simulink library "CryoDetLibCMB"  (R2016b)
settings: Solver=VariableStepAuto  StartTime=0.0  StopTime=10.0  RelTol=1e-3
undefined symbols (not defined in the file): A, B, C, D, Fadc, Fclk, PCIN, xlipgetpartsetting
libraries: xbsIndex_r4 x640, CryoDetLibCMB x81, CryoDetLib x2, simulink x1
(part 10 of 12)

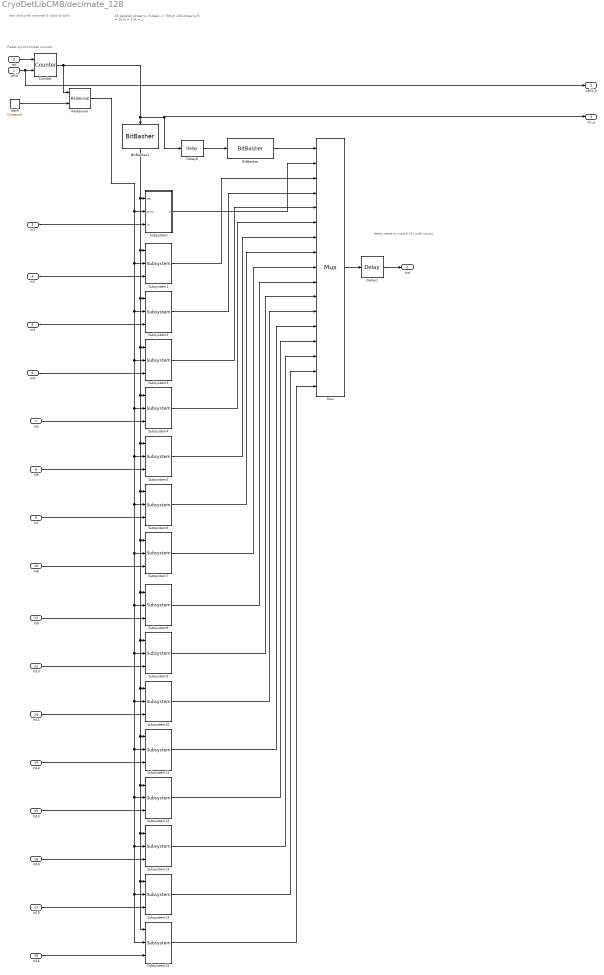
== system CryoDetLibCMB/decimate_128 ==
  note: 16 parallel streams, 8 deep -> TMUX 128 streams
      | R = 16
      | N = 3
      | M = 1
  note: Reset synchronizes counter
  note: set valid with channel 0 valid to sync
  note: delay need to match CH with inputs
  valid : Inport
  rst : Inport  Port=2
  In1 : Inport  Port=3
  In2 : Inport  Port=4
  In3 : Inport  Port=5
  In4 : Inport  Port=6
  In5 : Inport  Port=7
  In6 : Inport  Port=8
  In7 : Inport  Port=9
  In8 : Inport  Port=10
  In9 : Inport  Port=11
  In10 : Inport  Port=12
  In11 : Inport  Port=13
  In12 : Inport  Port=14
  In13 : Inport  Port=15
  In14 : Inport  Port=16
  In15 : Inport  Port=17
  In16 : Inport  Port=18
  BitBasher : xbsIndex_r4/BitBasher  bitexpr=sel = {cnt[3:0]}  display_expr=on  sr_1=sel  arith_type1=Unsigned  bin_pt1=0  sr_2=2  arith_type2=Unsigned  bin_pt2=0  sr_3=3  arith_type3=Unsigned  bin_pt3=0  sr_4=4  arith_type4=Unsigned  bin_pt4=0  dbl_ovrd=off  block_type=bitbasher
  BitBasher1 : xbsIndex_r4/BitBasher  bitexpr=sel = {cnt[6:4]}  display_expr=on  sr_1=sel  arith_type1=Unsigned  bin_pt1=0  sr_2=2  arith_type2=Unsigned  bin_pt2=0  sr_3=3  arith_type3=Unsigned  bin_pt3=0  sr_4=4  arith_type4=Unsigned  bin_pt4=0  dbl_ovrd=off  block_type=bitbasher
  Counter : xbsIndex_r4/Counter  cnt_type=Free Running  cnt_to=Inf  operation=Up  start_count=0  cnt_by_val=1  arith_type=Unsigned  n_bits=7  bin_pt=0  load_pin=off  rst=on  en=on  explicit_period=on  period=2/Fadc  use_behavioral_HDL=off  implementation=Fabric  dbl_ovrd=off  block_type=counter
  Delay1 : xbsIndex_r4/Delay  rst=off  infoeditControl=Selection of Reset will increase slice count due to use of real FFs and instead of SRLs  en=off  latency=14  reg_retiming=on  dbl_ovrd=off  block_type=delay
  Delay6 : xbsIndex_r4/Delay  rst=off  infoeditControl=Selection of Reset will increase slice count due to use of real FFs and instead of SRLs  en=off  latency=1  reg_retiming=on  dbl_ovrd=off  block_type=delay
  Mux : xbsIndex_r4/Mux  inputs=16  en=off  latency=1  precision=Full  arith_type=Unsigned  n_bits=16  bin_pt=14  quantization=Truncate  overflow=Wrap  dbl_ovrd=off  block_type=mux
  Relational : xbsIndex_r4/Relational  mode=a=b  op_type=Bool  en=off  latency=1  dbl_ovrd=off  block_type=relational
  Subsystem : Subsystem
  Subsystem{1..15} (15 alike) : CryoDetLibCMB/decimate_128/Subsystem
  latch : xbsIndex_r4/Constant  const=0  gui_display_data_type=Fixed-point  arith_type=Unsigned  n_bits=7  bin_pt=0  preci_type=Single  exp_width=8  frac_width=24  explicit_period=on  period=2/Fadc  equ=P=C  opselect=C  inp2=PCIN>>17  opr=+  inp1=P  carry=CIN  dbl_ovrd=off  block_type=constant
  valid_o : Outport
  out : Outport  Port=2
  ch_o : Outport  Port=3
  wires:
  rst/1 -> Counter/1
  Delay1/1 -> out/1
  valid/1 -> Counter/2, valid_o/1
  BitBasher1/1 -> Subsystem/1(sel), Subsystem1/1, Subsystem2/1, Subsystem3/1, Subsystem4/1, Subsystem5/1, Subsystem6/1, Subsystem7/1, Subsystem8/1, Subsystem9/1, Subsystem10/1, Subsystem11/1, Subsystem12/1, Subsystem13/1, Subsystem15/1, Subsystem14/1
  Counter/1 -> BitBasher1/1, Delay6/1, ch_o/1, Relational/1
  Subsystem3/1 -> Mux/5
  Mux/1 -> Delay1/1
  In16/1 -> Subsystem15/3
  In15/1 -> Subsystem14/3
  In14/1 -> Subsystem13/3
  In13/1 -> Subsystem12/3
  In12/1 -> Subsystem11/3
  In11/1 -> Subsystem10/3
  In10/1 -> Subsystem9/3
  In9/1 -> Subsystem8/3
  In8/1 -> Subsystem7/3
  In7/1 -> Subsystem6/3
  In6/1 -> Subsystem5/3
  In5/1 -> Subsystem4/3
  In4/1 -> Subsystem3/3
  In3/1 -> Subsystem2/3
  In2/1 -> Subsystem1/3
  In1/1 -> Subsystem/3(in)
  Subsystem15/1 -> Mux/17
  Subsystem14/1 -> Mux/16
  Subsystem13/1 -> Mux/15
  Subsystem12/1 -> Mux/14
  Subsystem11/1 -> Mux/13
  Subsystem10/1 -> Mux/12
  Subsystem9/1 -> Mux/11
  Subsystem8/1 -> Mux/10
  Subsystem7/1 -> Mux/9
  Subsystem6/1 -> Mux/8
  Subsystem5/1 -> Mux/7
  Subsystem4/1 -> Mux/6
  Subsystem2/1 -> Mux/4
  Subsystem1/1 -> Mux/3
  Subsystem/1(o) -> Mux/2
  BitBasher/1 -> Mux/1
  Relational/1 -> Subsystem/2(sync), Subsystem1/2, Subsystem2/2, Subsystem3/2, Subsystem4/2, Subsystem5/2, Subsystem6/2, Subsystem7/2, Subsystem8/2, Subsystem9/2, Subsystem10/2, Subsystem11/2, Subsystem12/2, Subsystem13/2, Subsystem15/2, Subsystem14/2
  latch/1 -> Relational/2
  Delay6/1 -> BitBasher/1

== system CryoDetLibCMB/demod 8Ch ==
  note: Scale by channel amplitude
  note: not tested yet!!!
  note: check scope for tlast errors
  note: Unity gain scaling is 2^-12
      | Here we add factor of 8 gain
      | assuming no single line is grater than -18 dBfs on ADC
  note: Should be 0 if prop delays adjusted properl
  note: compare subBand numbers to test for proper latency
      | diff should be zero otherwise adjust delay of suBand number to DDS block
  note: decimate by 16 3rd order
      | and adjust scaling appropriately
  note: Downconverter
  note: Multiply complex Signal & Reference
      | by complex LO and lowpass filter
      | send complex LO to:
      | 	DAC out
      | 	reference phase
      | ID is which demodulator is this one
  note: break out complex ADC signal
      | multiply by appropriate complex LO
      | then CIC decimate by 16
  note: first data comes out XX ticks after release of reset
  ID : Inport
  freqBus : Inport  Port=2
  In : Inport  Port=3
  amplBus : Inport  Port=4
  AddSub : xbsIndex_r4/AddSub  mode=Subtraction  use_carryin=off  use_carryout=off  en=off  latency=1  precision=User Defined  arith_type="Signed  (2's comp)"  n_bits=3  bin_pt=0  quantization=Truncate  overflow=Wrap  use_behavioral_HDL=off  hw_selection=Fabric  pipelined=off  dbl_ovrd=off  block_type=addsub
  Bus Creator1 : BusCreator  Inputs=4
  Bus Selector1 : BusSelector  OutputSignals=INDX,Q,I
  Bus Selector2 : BusSelector  OutputSignals=INDX,Q,I
  "CIC Compiler 4.0 " : xbsIndex_r4/CIC Compiler 4.0   filter_type=Decimation  number_of_stages=3  differential_delay=1  number_of_channels=8  sample_rate_changes=Fixed  fixed_or_initial_rate=16  minimum_rate=16  maximum_rate=16  ratespecification=Sample_Period  sampleperiod=1  hardwareoversamplingrate=1  quantization=Truncation  output_data_width=20  use_xtreme_dsp_slice=off  use_streaming_interface=on  has_aclken=off  has_aresetn=on  has_dout_tready=off  trim_axipin_name=on  gui_behaviour=Sysgen_GUI  input_data_width=18  ip_name=CIC Compiler  ip_version=4.0  dsptool_ready=true  wrapper_available=true  port_translation_map={ 'aclken' => 'en', 'aresetn' => 'rst' }  ipcore_xco_need_fpga_part=true  ipcore_verbose=false  block_type=cic_compiler_v4_0
  CIC Compiler 4.0 1 : xbsIndex_r4/CIC Compiler 4.0   filter_type=Decimation  number_of_stages=3  differential_delay=1  number_of_channels=8  sample_rate_changes=Fixed  fixed_or_initial_rate=16  minimum_rate=16  maximum_rate=16  ratespecification=Sample_Period  sampleperiod=1  hardwareoversamplingrate=1  quantization=Truncation  output_data_width=20  use_xtreme_dsp_slice=off  use_streaming_interface=on  has_aclken=off  has_aresetn=on  has_dout_tready=off  trim_axipin_name=on  gui_behaviour=Sysgen_GUI  input_data_width=18  ip_name=CIC Compiler  ip_version=4.0  dsptool_ready=true  wrapper_available=true  port_translation_map={ 'aclken' => 'en', 'aresetn' => 'rst' }  ipcore_xco_need_fpga_part=true  ipcore_verbose=false  block_type=cic_compiler_v4_0
  CIC debug scope : Scope  NumInputPorts=3
  CIC reset : Subsystem
  "Complex Multiplier 6.0 " : xbsIndex_r4/Complex Multiplier 6.0   hasatlast=off  hasatuser=on  atuserwidth=3  hasbtlast=off  hasbtuser=off  btuserwidth=1  multtype=Use_Mults  optimizegoal=Resources  flowcontrol=NonBlocking  outputwidth=18  roundmode=Truncate  hasctrltlast=off  hasctrltuser=off  ctrltuserwidth=1  outtlastbehv=Null  latencyconfig=Manual  minimumlatency=6  aclken=off  aresetn=off  trim_axipin_name=on  simulation_type=hybrid_sim  simulation_model=sysgen:cmpy_v6_0  data_path_portlist={ 's_axis_a_tdata_real', 's_axis_a_tdata_imag', 's_axis_b_tdata_real', 's_axis_b_tdata_imag', 's_axis_ctrl_tdata_rounding_bit', 'm_axis_dout_tdata_real', 'm_axis_dout_tdata_imag' }  aportwidth=63  bportwidth=63  ip_name=Complex Multiplier  ip_version=6.0  dsptool_ready=true  ipcore_usecache=true  ipcore_useipmodelcache=true  ipcore_verbose=false  ipcore_latency_parameter='minimumlatency'  wrapper_available=true  port_translation_map={ 'aclken' => 'en', 'aresetn' => 'rst'}  block_type=cmpy_v6_0
  Constant : xbsIndex_r4/Constant  const=1  gui_display_data_type=Boolean  arith_type=Boolean  n_bits=16  bin_pt=14  preci_type=Single  exp_width=8  frac_width=24  explicit_period=off  period=1  equ=P=C  opselect=C  inp2=PCIN>>17  opr=+  inp1=P  carry=CIN  dbl_ovrd=off  block_type=constant
  Constant1 : xbsIndex_r4/Constant  const=1  gui_display_data_type=Boolean  arith_type=Boolean  n_bits=16  bin_pt=14  preci_type=Single  exp_width=8  frac_width=24  explicit_period=off  period=1  equ=P=C  opselect=C  inp2=PCIN>>17  opr=+  inp1=P  carry=CIN  dbl_ovrd=off  block_type=constant
  Constant4 : xbsIndex_r4/Constant  const=14  gui_display_data_type=Fixed-point  arith_type=Unsigned  n_bits=4  bin_pt=0  preci_type=Single  exp_width=8  frac_width=24  explicit_period=off  period=1  equ=P=C  opselect=C  inp2=PCIN>>17  opr=+  inp1=P  carry=CIN  dbl_ovrd=off  block_type=constant
  DDS 8ch : Subsystem
  Delay1 : xbsIndex_r4/Delay  rst=off  infoeditControl=Selection of Reset will increase slice count due to use of real FFs and instead of SRLs  en=off  latency=1  reg_retiming=on  dbl_ovrd=off  block_type=delay
  Delay5 : xbsIndex_r4/Delay  rst=off  infoeditControl=Selection of Reset will increase slice count due to use of real FFs and instead of SRLs  en=off  latency=1  reg_retiming=on  dbl_ovrd=off  block_type=delay
  Delay6 : xbsIndex_r4/Delay  rst=off  infoeditControl=Selection of Reset will increase slice count due to use of real FFs and instead of SRLs  en=off  latency=1  reg_retiming=on  dbl_ovrd=off  block_type=delay
  Display : Display
  Gateway Out{,1..5} (6 alike) : xbsIndex_r4/Gateway Out  inherit_from_input=off  hdl_port=off  rows=1  columns=1  UseAsDAC=off  DACChannel='1'  interface=None  automatic_assignment=on  address_offset=hex2dec('00')  intf_name=''  intf_description=''  timing_constraint=None  locs_specified=off  LOCs={}  io_standard={}  block_type=gatewayout
  Mux : Mux  Inputs=2
  Mux1 : Mux  Inputs=2
  Scale1 : xbsIndex_r4/Scale  scale_factor=-9  dbl_ovrd=off  block_type=scale
  Scale2 : xbsIndex_r4/Scale  scale_factor=-9  dbl_ovrd=off  block_type=scale
  Set Ampls : Subsystem
  Terminator1 : Terminator
  Terminator2 : Terminator
  Terminator3 : Terminator
  phaseRefDownsample : Subsystem
  demod : Outport
  phase ref : Outport  Port=2
  tones out : Outport  Port=3
  wires:
  In/1 -> Bus Selector2/1
  Bus Selector1/2 -> "Complex Multiplier 6.0 "/2  "<Q>"
  Bus Selector1/3 -> "Complex Multiplier 6.0 "/3  "<I>"
  "Complex Multiplier 6.0 "/2 -> "CIC Compiler 4.0 "/2
  "CIC Compiler 4.0 "/3 -> Scale1/1
  CIC Compiler 4.0 1/3 -> Scale2/1
  "CIC Compiler 4.0 "/1 -> Terminator1/1
  CIC Compiler 4.0 1/1 -> Terminator2/1
  CIC Compiler 4.0 1/2 -> Terminator3/1
  "Complex Multiplier 6.0 "/3 -> CIC Compiler 4.0 1/2
  Constant/1 -> "Complex Multiplier 6.0 "/5, "Complex Multiplier 6.0 "/1
  ID/1 -> DDS 8ch/1(ID), [ID]
  freqBus/1 -> DDS 8ch/2(freqBus)
  Bus Selector2/1 -> Delay1/1, DDS 8ch/3(band)  "<INDX>"
  Bus Selector2/2 -> Delay5/1  "<Q>"
  Bus Selector2/3 -> Delay6/1  "<I>"
  DDS 8ch/1(IQ out) -> tones out/1, Bus Selector1/1
  Delay1/1 -> AddSub/2, "Complex Multiplier 6.0 "/4
  Delay5/1 -> "Complex Multiplier 6.0 "/6
  Delay6/1 -> "Complex Multiplier 6.0 "/7
  Bus Selector1/1 -> AddSub/1  "<INDX>"
  AddSub/1 -> Gateway Out/1
  Gateway Out/1 -> Display/1
  Constant1/1 -> CIC Compiler 4.0 1/1, "CIC Compiler 4.0 "/1
  Constant4/1 -> CIC reset/3(N-2)
  [fpgaReset] -> CIC reset/1(resetIn)
  CIC reset/1(notResetOut) -> "CIC Compiler 4.0 "/4, CIC Compiler 4.0 1/4
  "Complex Multiplier 6.0 "/4 -> CIC reset/2(Channel)
  CIC reset/2(tlast) -> CIC Compiler 4.0 1/3, "CIC Compiler 4.0 "/3
  "CIC Compiler 4.0 "/6 -> Bus Creator1/2  "band"
  Scale1/1 -> Bus Creator1/3  "Q"
  Scale2/1 -> Bus Creator1/4  "I"
  CIC Compiler 4.0 1/4 -> Gateway Out1/1
  CIC Compiler 4.0 1/5 -> phaseRefDownsample/2(chanSynch), Gateway Out2/1
  CIC Compiler 4.0 1/6 -> Gateway Out3/1
  CIC Compiler 4.0 1/7 -> Gateway Out4/1
  CIC Compiler 4.0 1/8 -> Gateway Out5/1
  Gateway Out2/1 -> Mux/2
  Gateway Out1/1 -> Mux/1
  Gateway Out5/1 -> Mux1/2
  Gateway Out4/1 -> Mux1/1
  Mux/1 -> CIC debug scope/1
  Gateway Out3/1 -> CIC debug scope/2
  Mux1/1 -> CIC debug scope/3
  "CIC Compiler 4.0 "/2 -> Bus Creator1/1  "tvalid"
  DDS 8ch/2(phaseRef out) -> phaseRefDownsample/1(In1)
  phaseRefDownsample/1(Out1) -> phase ref/1
  Bus Creator1/1 -> Set Ampls/3(DDS IQ)
  Set Ampls/1(IQ out) -> demod/1
  [ID] -> Set Ampls/1(ID)
  amplBus/1 -> Set Ampls/2(amplBus)

== system CryoDetLibCMB/demod setup stuff ==
  Bus Creator : BusCreator  Inputs=3
  Bus Creator1 : BusCreator  Inputs=3
  Counter Free-Running1 : simulink/Sources/Counter Free-Running  NumBits=3  tsamp=Tclk
  I : xbsIndex_r4/Constant  const=1  gui_display_data_type=Fixed-point  arith_type=Signed (2's comp)  n_bits=25  bin_pt=24  preci_type=Single  exp_width=8  frac_width=24  explicit_period=on  period=Tclk  equ=P=C  opselect=C  inp2=PCIN>>17  opr=+  inp1=P  carry=CIN  dbl_ovrd=off  block_type=constant
  Ndemod : xbsIndex_r4/Constant  const=15  gui_display_data_type=Fixed-point  arith_type=Unsigned  n_bits=4  bin_pt=0  preci_type=Single  exp_width=8  frac_width=24  explicit_period=off  period=1  equ=P=C  opselect=C  inp2=PCIN>>17  opr=+  inp1=P  carry=CIN  dbl_ovrd=off  block_type=constant
  Q : xbsIndex_r4/Constant  const=0  gui_display_data_type=Fixed-point  arith_type=Signed (2's comp)  n_bits=25  bin_pt=24  preci_type=Single  exp_width=8  frac_width=24  explicit_period=on  period=Tclk  equ=P=C  opselect=C  inp2=PCIN>>17  opr=+  inp1=P  carry=CIN  dbl_ovrd=off  block_type=constant
  demod # : xbsIndex_r4/Constant  const=15  gui_display_data_type=Fixed-point  arith_type=Unsigned  n_bits=4  bin_pt=0  preci_type=Single  exp_width=8  frac_width=24  explicit_period=off  period=1  equ=P=C  opselect=C  inp2=PCIN>>17  opr=+  inp1=P  carry=CIN  dbl_ovrd=off  block_type=constant
  freq2 : xbsIndex_r4/Constant  const=0.12345 * 2^24  gui_display_data_type=Fixed-point  arith_type=Unsigned  n_bits=24  bin_pt=0  preci_type=Single  exp_width=8  frac_width=24  explicit_period=on  period=Tclk  equ=P=C  opselect=C  inp2=PCIN>>17  opr=+  inp1=P  carry=CIN  dbl_ovrd=off  block_type=constant
  subCh : xbsIndex_r4/Constant  const=7  gui_display_data_type=Fixed-point  arith_type=Unsigned  n_bits=3  bin_pt=0  preci_type=Single  exp_width=8  frac_width=24  explicit_period=off  period=1  equ=P=C  opselect=C  inp2=PCIN>>17  opr=+  inp1=P  carry=CIN  dbl_ovrd=off  block_type=constant
  demod numberl : Outport
  freqBus : Outport  Port=2
  subBandIQ : Outport  Port=3
  wires:
  Bus Creator/1 -> freqBus/1
  demod #/1 -> demod numberl/1
  freq2/1 -> Bus Creator/3  "freq"
  subCh/1 -> Bus Creator/1  "band"
  Ndemod/1 -> Bus Creator/2  "chan"
  Bus Creator1/1 -> subBandIQ/1
  Counter Free-Running1/1 -> Bus Creator1/1  "INDX"
  Q/1 -> Bus Creator1/2  "Q"
  I/1 -> Bus Creator1/3  "I"

== system CryoDetLibCMB/freqWordDecoder ==
  Fi : Inport
  BitBasher : xbsIndex_r4/BitBasher  bitexpr=|  display_expr=on  sr_1=FBen  arith_type1=Unsigned  bin_pt1=0  sr_2=ampl  arith_type2=Unsigned  bin_pt2=0  sr_3=Finit  arith_type3=Unsigned  bin_pt3=24  sr_4=4  arith_type4=Unsigned  bin_pt4=0  dbl_ovrd=off  block_type=bitbasher
      | FBen = {freqWord[31:31]}
      | ampl = {freqWord[27:24]}
      | Finit = {freqWord[23:0]}
  FBen : Outport
  ampl : Outport  Port=2
  Fc : Outport  Port=3
  wires:
  BitBasher/2 -> ampl/1
  BitBasher/3 -> Fc/1
  BitBasher/1 -> FBen/1
  Fi/1 -> BitBasher/1

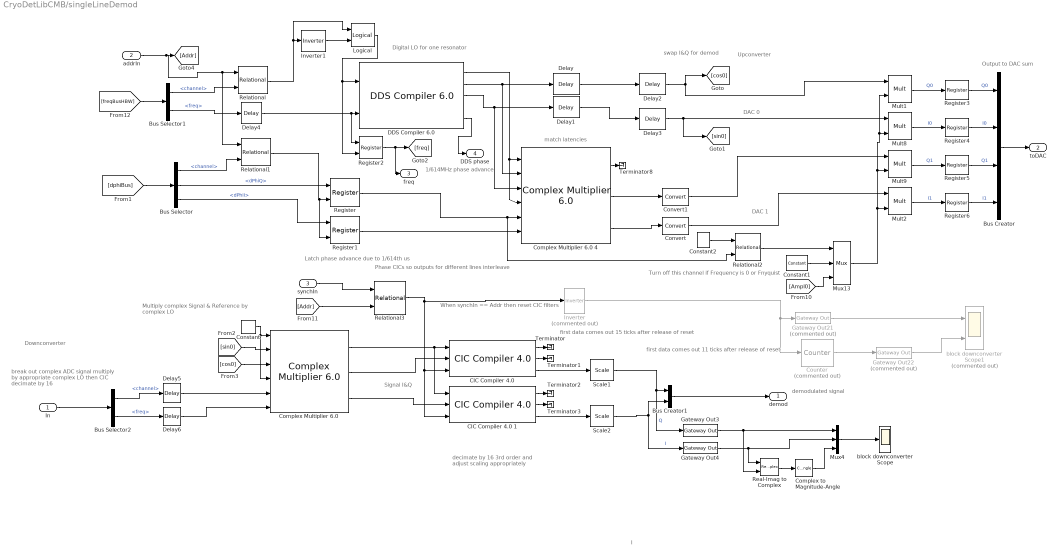
== system CryoDetLibCMB/singleLineDemod ==
  note: swap I&Q for demod
  note: Output to DAC sum
  note: decimate by 16 3rd order
      | and adjust scaling appropriately
  note: When synchIn == Addr then reset CIC filters
  note: Turn off this channel if Frequency is 0 or Fnyquist
  note: first data comes out 15 ticks after release of reset
  note: Latch phase advance due to 1/614th us
  note: I
  note: DAC 1
  note: DAC 0
  note: Downconverter
  note: demodulated signal
  note: Phase CICs so outputs for different lines interleave
  note: Signal I&Q
  note: Multiply complex Signal & Reference
      | by complex LO
  note: match latencies
  note: 1/614MHz
      | phase advance
  note: break out complex ADC signal
      | multiply by appropriate complex LO
      | then CIC decimate by 16
  note: Digital LO for one resonator
  note: Upconverter
  note: first data comes out 11 ticks after release of reset
  In : Inport
  addrIn : Inport  Port=2
  synchIn : Inport  Port=3
  Bus Creator : BusCreator  Inputs=4
  Bus Creator1 : BusCreator  Inputs=2
  Bus Selector : BusSelector  OutputSignals=channel,dPhiQ,dPhiI
  Bus Selector1 : BusSelector  OutputSignals=channel,freq
  Bus Selector2 : BusSelector  OutputSignals=channel,freq
  "CIC Compiler 4.0 " : xbsIndex_r4/CIC Compiler 4.0   filter_type=Decimation  number_of_stages=3  differential_delay=1  number_of_channels=1  sample_rate_changes=Fixed  fixed_or_initial_rate=16  minimum_rate=16  maximum_rate=16  ratespecification=Sample_Period  sampleperiod=1  hardwareoversamplingrate=1  quantization=Truncation  output_data_width=20  use_xtreme_dsp_slice=off  use_streaming_interface=on  has_aclken=off  has_aresetn=on  has_dout_tready=off  trim_axipin_name=on  gui_behaviour=Sysgen_GUI  input_data_width=18  ip_name=CIC Compiler  ip_version=4.0  dsptool_ready=true  wrapper_available=true  port_translation_map={ 'aclken' => 'en', 'aresetn' => 'rst' }  ipcore_xco_need_fpga_part=true  ipcore_verbose=false  block_type=cic_compiler_v4_0
  CIC Compiler 4.0 1 : xbsIndex_r4/CIC Compiler 4.0   filter_type=Decimation  number_of_stages=3  differential_delay=1  number_of_channels=1  sample_rate_changes=Fixed  fixed_or_initial_rate=16  minimum_rate=16  maximum_rate=16  ratespecification=Sample_Period  sampleperiod=1  hardwareoversamplingrate=1  quantization=Truncation  output_data_width=20  use_xtreme_dsp_slice=off  use_streaming_interface=on  has_aclken=off  has_aresetn=on  has_dout_tready=off  trim_axipin_name=on  gui_behaviour=Sysgen_GUI  input_data_width=18  ip_name=CIC Compiler  ip_version=4.0  dsptool_ready=true  wrapper_available=true  port_translation_map={ 'aclken' => 'en', 'aresetn' => 'rst' }  ipcore_xco_need_fpga_part=true  ipcore_verbose=false  block_type=cic_compiler_v4_0
  "Complex Multiplier 6.0 " : xbsIndex_r4/Complex Multiplier 6.0   hasatlast=off  hasatuser=off  atuserwidth=1  hasbtlast=off  hasbtuser=off  btuserwidth=1  multtype=Use_Mults  optimizegoal=Resources  flowcontrol=NonBlocking  outputwidth=18  roundmode=Truncate  hasctrltlast=off  hasctrltuser=off  ctrltuserwidth=1  outtlastbehv=Null  latencyconfig=Automatic  minimumlatency=37  aclken=off  aresetn=off  trim_axipin_name=on  simulation_type=hybrid_sim  simulation_model=sysgen:cmpy_v6_0  data_path_portlist={ 's_axis_a_tdata_real', 's_axis_a_tdata_imag', 's_axis_b_tdata_real', 's_axis_b_tdata_imag', 's_axis_ctrl_tdata_rounding_bit', 'm_axis_dout_tdata_real', 'm_axis_dout_tdata_imag' }  aportwidth=63  bportwidth=63  ip_name=Complex Multiplier  ip_version=6.0  dsptool_ready=true  ipcore_usecache=true  ipcore_useipmodelcache=true  ipcore_verbose=false  ipcore_latency_parameter='minimumlatency'  wrapper_available=true  port_translation_map={ 'aclken' => 'en', 'aresetn' => 'rst'}  block_type=cmpy_v6_0
  Complex Multiplier 6.0 4 : xbsIndex_r4/Complex Multiplier 6.0   hasatlast=off  hasatuser=off  atuserwidth=1  hasbtlast=off  hasbtuser=off  btuserwidth=1  multtype=Use_Mults  optimizegoal=Resources  flowcontrol=NonBlocking  outputwidth=19  roundmode=Truncate  hasctrltlast=off  hasctrltuser=off  ctrltuserwidth=1  outtlastbehv=Null  latencyconfig=Manual  minimumlatency=6  aclken=off  aresetn=off  trim_axipin_name=on  simulation_type=hybrid_sim  simulation_model=sysgen:cmpy_v6_0  data_path_portlist={ 's_axis_a_tdata_real', 's_axis_a_tdata_imag', 's_axis_b_tdata_real', 's_axis_b_tdata_imag', 's_axis_ctrl_tdata_rounding_bit', 'm_axis_dout_tdata_real', 'm_axis_dout_tdata_imag' }  aportwidth=63  bportwidth=63  ip_name=Complex Multiplier  ip_version=6.0  dsptool_ready=true  ipcore_usecache=true  ipcore_useipmodelcache=true  ipcore_verbose=false  ipcore_latency_parameter='minimumlatency'  wrapper_available=true  port_translation_map={ 'aclken' => 'en', 'aresetn' => 'rst'}  block_type=cmpy_v6_0
  Complex to Magnitude-Angle : ComplexToMagnitudeAngle  Output=Magnitude
  Constant : xbsIndex_r4/Constant  const=1  gui_display_data_type=Boolean  arith_type=Boolean  n_bits=16  bin_pt=14  preci_type=Single  exp_width=8  frac_width=24  explicit_period=off  period=1  equ=P=C  opselect=C  inp2=PCIN>>17  opr=+  inp1=P  carry=CIN  dbl_ovrd=off  block_type=constant
  Constant1 : xbsIndex_r4/Constant  const=0  gui_display_data_type=Fixed-point  arith_type=Unsigned  n_bits=16  bin_pt=16  preci_type=Single  exp_width=8  frac_width=24  explicit_period=off  period=1  equ=P=C  opselect=C  inp2=PCIN>>17  opr=+  inp1=P  carry=CIN  dbl_ovrd=off  block_type=constant
  Constant2 : xbsIndex_r4/Constant  const=0  gui_display_data_type=Fixed-point  arith_type=Unsigned  n_bits=16  bin_pt=16  preci_type=Single  exp_width=8  frac_width=24  explicit_period=off  period=1  equ=P=C  opselect=C  inp2=PCIN>>17  opr=+  inp1=P  carry=CIN  dbl_ovrd=off  block_type=constant
  Convert : xbsIndex_r4/Convert  gui_display_data_type=Fixed-point  arith_type="Signed  (2's comp)"  n_bits=16  bin_pt=14  float_type=Single  exp_bits=8  fraction_bits=24  quantization=Truncate  overflow=Saturate  en=off  latency=1  pipeline=off  dbl_ovrd=off  block_type=convert
  Convert1 : xbsIndex_r4/Convert  gui_display_data_type=Fixed-point  arith_type="Signed  (2's comp)"  n_bits=16  bin_pt=14  float_type=Single  exp_bits=8  fraction_bits=24  quantization=Truncate  overflow=Saturate  en=off  latency=1  pipeline=off  dbl_ovrd=off  block_type=convert
  Counter : xbsIndex_r4/Counter  Commented=on  cnt_type=Free Running  cnt_to=Inf  operation=Up  start_count=0  cnt_by_val=2^-8  arith_type=Unsigned  n_bits=8  bin_pt=8  load_pin=off  rst=on  en=off  explicit_period=off  period=1  use_behavioral_HDL=off  implementation=Fabric  dbl_ovrd=off  block_type=counter
  "DDS Compiler 6.0 " : xbsIndex_r4/DDS Compiler 6.0   partspresent=Phase_Generator_and_SIN_COS_LUT  dds_clock_rate=Fclk/1e6  channels=1  mode_of_operation=Standard  modulus=9  parameter_entry=Hardware_Parameters  spurious_free_dynamic_range=45  frequency_resolution=0.4  noise_shaping=None  phase_width=freqBits  output_width=IQbits  output_selection=Sine_and_Cosine  negative_sine=off  negative_cosine=off  amplitude_mode=Unit_Circle  memory_type=Auto  optimization_goal=Speed  dsp48_use=Maximal  resync=off  latency_configuration=Configurable  latency=15  has_phase_out=on  has_aclken=off  has_aresetn=off  explicit_period=on  period=Tclk  data_has_tlast=Not_Required  has_tready=off  s_phase_has_tuser=Not_Required  m_data_has_tuser=Not_Required  m_phase_has_tuser=Not_Required  s_phase_tuser_width=1  output_form=Twos_Complement  s_config_sync_mode=On_Vector  phase_increment=Programmable  output_frequency1=0  output_frequency2=0  output_frequency3=0  output_frequency4=0  output_frequency5=0  output_frequency6=0  output_frequency7=0  output_frequency8=0  output_frequency9=0  output_frequency10=0  output_frequency11=0  output_frequency12=0  output_frequency13=0  output_frequency14=0  output_frequency15=0  output_frequency16=0  pinc1='0'  pinc2='0'  pinc3='0'  pinc4='0'  pinc5='0'  pinc6='0'  pinc7='0'  pinc8='0'  pinc9='0'  pinc10='0'  pinc11='0'  pinc12='0'  pinc13='0'  pinc14='0'  pinc15='0'  pinc16='0'  phase_offset=None  phase_offset_angles1=0  phase_offset_angles2=0  phase_offset_angles3=0  phase_offset_angles4=0  phase_offset_angles5=0  phase_offset_angles6=0  phase_offset_angles7=0  phase_offset_angles8=0  phase_offset_angles9=0  phase_offset_angles10=0  phase_offset_angles11=0  phase_offset_angles12=0  phase_offset_angles13=0  phase_offset_angles14=0  phase_offset_angles15=0  phase_offset_angles16=0  poff1='0'  poff2='0'  poff3='0'  poff4='0'  poff5='0'  poff6='0'  poff7='0'  poff8='0'  poff9='0'  poff10='0'  poff11='0'  poff12='0'  poff13='0'  poff14='0'  poff15='0'  poff16='0'  trim_axipin_name=on  simulation_type=hybrid_sim  simulation_model=sysgen:xddsv6_0_cmodel  data_path_portlist={ 's_axis_config_tdata_poff', 's_axis_config_tdata_chan0_poff', 's_axis_config_tdata_pinc', 's_axis_config_tdata_chan0_pinc', 's_axis_phase_tdata_resync', 's_axis_phase_tdata_chan0_resync', 's_axis_phase_tdata_poff', 's_axis_phase_tdata_chan0_poff', 's_axis_phase_tdata_pinc', 's_axis_phase_tdata_chan0_pinc', 's_axis_phase_tdata_phase_in', 'm_axis_data_tdata_sine', 'm_axis_data_tdata_chan0_sine', 'm_axis_data_tdata_cosine', 'm_axis_data_tdata_chan0_cosine', 'm_axis_phase_tdata_phase_out', 'm_axis_phase_tdata_chan0_phase_out'}  por_mode=false  gui_behaviour=Sysgen  ip_name=DDS Compiler  ip_version=6.0  dsptool_ready=true  wrapper_available=true  port_translation_map={ 'aclken' => 'en', 'aresetn' => 'rst' }  ipcore_usecache=true  ipcore_useipmodelcache=true  ipcore_xco_need_fpga_part=true  ipcore_fpga_part=xlipgetpartsetting(gcb, {'kintex7', 'xc7k325t', '-3', 'fbg676'})  ipcore_verbose=false  block_type=dds_compiler_v6_0
  Delay : xbsIndex_r4/Delay  rst=off  infoeditControl=Selection of Reset will increase slice count due to use of real FFs and instead of SRLs  en=off  latency=6  reg_retiming=off  dbl_ovrd=off  block_type=delay
  Delay1 : xbsIndex_r4/Delay  rst=off  infoeditControl=Selection of Reset will increase slice count due to use of real FFs and instead of SRLs  en=off  latency=6  reg_retiming=off  dbl_ovrd=off  block_type=delay
  Delay2 : xbsIndex_r4/Delay  rst=off  infoeditControl=Selection of Reset will increase slice count due to use of real FFs and instead of SRLs  en=off  latency=1  reg_retiming=off  dbl_ovrd=off  block_type=delay
  Delay3 : xbsIndex_r4/Delay  rst=off  infoeditControl=Selection of Reset will increase slice count due to use of real FFs and instead of SRLs  en=off  latency=1  reg_retiming=off  dbl_ovrd=off  block_type=delay
  Delay4 : xbsIndex_r4/Delay  rst=off  infoeditControl=Selection of Reset will increase slice count due to use of real FFs and instead of SRLs  en=off  latency=2  reg_retiming=on  dbl_ovrd=off  block_type=delay
  Delay5 : xbsIndex_r4/Delay  rst=off  infoeditControl=Selection of Reset will increase slice count due to use of real FFs and instead of SRLs  en=off  latency=2  reg_retiming=on  dbl_ovrd=off  block_type=delay
  Delay6 : xbsIndex_r4/Delay  rst=off  infoeditControl=Selection of Reset will increase slice count due to use of real FFs and instead of SRLs  en=off  latency=2  reg_retiming=on  dbl_ovrd=off  block_type=delay
  Gateway Out21 : xbsIndex_r4/Gateway Out  Commented=on  inherit_from_input=off  hdl_port=off  rows=1  columns=1  UseAsDAC=off  DACChannel='1'  interface=None  automatic_assignment=on  address_offset=hex2dec('00')  intf_name=''  intf_description=''  timing_constraint=None  locs_specified=off  LOCs={}  io_standard={}  block_type=gatewayout
  Gateway Out22 : xbsIndex_r4/Gateway Out  Commented=on  inherit_from_input=off  hdl_port=off  rows=1  columns=1  UseAsDAC=off  DACChannel='1'  interface=None  automatic_assignment=on  address_offset=hex2dec('00')  intf_name=''  intf_description=''  timing_constraint=None  locs_specified=off  LOCs={}  io_standard={}  block_type=gatewayout
  Gateway Out3 : xbsIndex_r4/Gateway Out  inherit_from_input=off  hdl_port=off  rows=1  columns=1  UseAsDAC=off  DACChannel='1'  interface=None  automatic_assignment=on  address_offset=hex2dec('00')  intf_name=''  intf_description=''  timing_constraint=None  locs_specified=off  LOCs={}  io_standard={}  block_type=gatewayout
  Gateway Out4 : xbsIndex_r4/Gateway Out  inherit_from_input=off  hdl_port=off  rows=1  columns=1  UseAsDAC=off  DACChannel='1'  interface=None  automatic_assignment=on  address_offset=hex2dec('00')  intf_name=''  intf_description=''  timing_constraint=None  locs_specified=off  LOCs={}  io_standard={}  block_type=gatewayout
  Inverter : xbsIndex_r4/Inverter  Commented=on  en=off  latency=0  dbl_ovrd=off  block_type=inv
  Inverter1 : xbsIndex_r4/Inverter  en=off  latency=1  dbl_ovrd=off  block_type=inv
  Logical : xbsIndex_r4/Logical  logical_function=AND  inputs=2  en=off  latency=1  precision=Full  arith_type=Unsigned  n_bits=16  bin_pt=0  align_bp=on  dbl_ovrd=off  block_type=logical
  Mult{1..2,8..9} (4 alike) : xbsIndex_r4/Mult  precision=User Defined  arith_type="Signed  (2's comp)"  n_bits=16  bin_pt=15  quantization=Truncate  overflow=Wrap  en=off  latency=3  use_behavioral_HDL=off  opt=Speed  use_embedded=on  optimum_pipeline=off  pipeline=on  dbl_ovrd=off  use_rpm=on  placement_style=Triangular  block_type=mult
  Mux13 : xbsIndex_r4/Mux  inputs=2  en=off  latency=0  precision=Full  arith_type=Unsigned  n_bits=16  bin_pt=14  quantization=Truncate  overflow=Wrap  dbl_ovrd=off  block_type=mux
  Mux4 : Mux  Inputs=3
  Real-Imag to Complex : RealImagToComplex
  Register : xbsIndex_r4/Register  init=0  rst=off  en=on  dbl_ovrd=off  block_type=register
  Register1 : xbsIndex_r4/Register  init=0  rst=off  en=on  dbl_ovrd=off  block_type=register
  Register2 : xbsIndex_r4/Register  init=0  rst=off  en=on  dbl_ovrd=off  block_type=register
  Register{3..6} (4 alike) : xbsIndex_r4/Register  init=0  rst=off  en=off  dbl_ovrd=off  block_type=register
  Relational : xbsIndex_r4/Relational  mode=a=b  op_type=Bool  en=off  latency=1  dbl_ovrd=off  block_type=relational
  Relational1 : xbsIndex_r4/Relational  mode=a=b  op_type=Bool  en=off  latency=0  dbl_ovrd=off  block_type=relational
  Relational2 : xbsIndex_r4/Relational  mode=a!=b  op_type=Ufix  en=off  latency=1  dbl_ovrd=off  block_type=relational
  Relational3 : xbsIndex_r4/Relational  mode=a!=b  op_type=Bool  en=off  latency=0  dbl_ovrd=off  block_type=relational
  Scale1 : xbsIndex_r4/Scale  scale_factor=-12  dbl_ovrd=off  block_type=scale
  Scale2 : xbsIndex_r4/Scale  scale_factor=-12  dbl_ovrd=off  block_type=scale
  Terminator{,1..3,8} (5 alike) : Terminator
  block downconverter Scope : Scope
  block downconverter Scope1 : Scope  Commented=on  NumInputPorts=2
  demod : Outport
  toDAC : Outport  Port=2
  freq : Outport  Port=3
  DDS phase : Outport  Port=4
  wires:
  Relational/1 -> Logical/1, Inverter1/1
  Bus Selector1/1 -> Relational/2  "<channel>"
  Bus Selector1/2 -> Delay4/1  "<freq>"
  addrIn/1 -> Relational1/1, Relational/1, [Addr]
  "DDS Compiler 6.0 "/2 -> Complex Multiplier 6.0 4/2, Delay/1
  "DDS Compiler 6.0 "/3 -> Complex Multiplier 6.0 4/3, Delay1/1
  In/1 -> Bus Selector2/1
  Relational1/1 -> Register1/2, Register/2
  Register1/1 -> Complex Multiplier 6.0 4/6
  Register/1 -> Relational2/2, Complex Multiplier 6.0 4/5
  "DDS Compiler 6.0 "/1 -> Complex Multiplier 6.0 4/1, Complex Multiplier 6.0 4/4
  Delay/1 -> Delay2/1
  Delay1/1 -> Delay3/1
  [sin0] -> "Complex Multiplier 6.0 "/2
  [cos0] -> "Complex Multiplier 6.0 "/3
  "Complex Multiplier 6.0 "/2 -> "CIC Compiler 4.0 "/2
  "CIC Compiler 4.0 "/3 -> Scale1/1
  CIC Compiler 4.0 1/3 -> Scale2/1
  "Complex Multiplier 6.0 "/1 -> "CIC Compiler 4.0 "/1, CIC Compiler 4.0 1/1
  "CIC Compiler 4.0 "/1 -> Terminator/1
  CIC Compiler 4.0 1/1 -> Terminator2/1
  CIC Compiler 4.0 1/2 -> Terminator3/1
  Complex Multiplier 6.0 4/1 -> Terminator8/1
  Bus Creator/1 -> toDAC/1
  Bus Selector/2 -> Register/1  "<dPhiQ>"
  Bus Selector/3 -> Register1/1  "<dPhiI>"
  [dphiBus] -> Bus Selector/1
  Bus Selector/1 -> Relational1/2  "<channel>"
  Complex Multiplier 6.0 4/3 -> Convert/1
  Complex Multiplier 6.0 4/2 -> Convert1/1
  Constant1/1 -> Mux13/2
  [Ampl0] -> Mux13/3
  Mux13/1 -> Mult2/2, Mult9/2, Mult1/2, Mult8/2
  Constant2/1 -> Relational2/1
  Relational2/1 -> Mux13/1
  Relational3/1 -> Inverter/1, CIC Compiler 4.0 1/3, "CIC Compiler 4.0 "/3
  [Addr] -> Relational3/2
  synchIn/1 -> Relational3/1
  "CIC Compiler 4.0 "/2 -> Terminator1/1
  [freqBusHBW] -> Bus Selector1/1
  Convert1/1 -> Mult9/1
  Delay3/1 -> [sin0], Mult8/1
  Delay2/1 -> Mult1/1, [cos0]
  Delay4/1 -> Register2/1, "DDS Compiler 6.0 "/2
  Inverter1/1 -> Logical/2
  Logical/1 -> Register2/2, "DDS Compiler 6.0 "/1
  "Complex Multiplier 6.0 "/3 -> CIC Compiler 4.0 1/2
  Constant/1 -> "Complex Multiplier 6.0 "/4, "Complex Multiplier 6.0 "/1
  Convert/1 -> Mult2/1
  Mult2/1 -> Register6/1  "I1"
  Mult9/1 -> Register5/1  "Q1"
  Mult8/1 -> Register4/1  "I0"
  Mult1/1 -> Register3/1  "Q0"
  Bus Creator1/1 -> demod/1
  Scale1/1 -> Gateway Out3/1, Bus Creator1/1  "Q"
  Scale2/1 -> Gateway Out4/1, Bus Creator1/2  "I"
  Gateway Out4/1 -> Mux4/2, Real-Imag to Complex/1
  Gateway Out3/1 -> Mux4/1, Real-Imag to Complex/2
  Mux4/1 -> block downconverter Scope/1
  Gateway Out22/1 -> block downconverter Scope1/2
  Complex to Magnitude-Angle/1 -> Mux4/3
  Gateway Out21/1 -> block downconverter Scope1/1
  Counter/1 -> Gateway Out22/1
  Inverter/1 -> Counter/1, Gateway Out21/1
  Real-Imag to Complex/1 -> Complex to Magnitude-Angle/1
  Register2/1 -> freq/1, [freq]
  Delay6/1 -> "Complex Multiplier 6.0 "/6
  Delay5/1 -> "Complex Multiplier 6.0 "/5
  Register3/1 -> Bus Creator/1  "Q0"
  Register4/1 -> Bus Creator/2  "I0"
  Register5/1 -> Bus Creator/3  "Q1"
  Register6/1 -> Bus Creator/4  "I1"
  "DDS Compiler 6.0 "/5 -> DDS phase/1
  Bus Selector2/2 -> Delay6/1  "<freq>"
  Bus Selector2/1 -> Delay5/1  "<channel>"

== system CryoDetLibCMB/tmux_integrator ==
  sel : Inport
  sync : Inport  Port=2
  in : Inport  Port=3
  AddSub : xbsIndex_r4/AddSub  mode=Addition  use_carryin=off  use_carryout=off  en=off  latency=3  precision=User Defined  arith_type="Signed  (2's comp)"  n_bits=n_bit  bin_pt=b_pt  quantization=Truncate  overflow=Wrap  use_behavioral_HDL=on  hw_selection=Fabric  pipelined=off  dbl_ovrd=off  block_type=addsub
  AddSub1 : xbsIndex_r4/AddSub  mode=Addition  use_carryin=off  use_carryout=off  en=off  latency=3  precision=User Defined  arith_type="Signed  (2's comp)"  n_bits=n_bit  bin_pt=b_pt  quantization=Truncate  overflow=Wrap  use_behavioral_HDL=on  hw_selection=Fabric  pipelined=off  dbl_ovrd=off  block_type=addsub
  AddSub2 : xbsIndex_r4/AddSub  mode=Addition  use_carryin=off  use_carryout=off  en=off  latency=3  precision=User Defined  arith_type="Signed  (2's comp)"  n_bits=n_bit  bin_pt=b_pt  quantization=Truncate  overflow=Wrap  use_behavioral_HDL=on  hw_selection=Fabric  pipelined=off  dbl_ovrd=off  block_type=addsub
  Delay : xbsIndex_r4/Delay  rst=off  infoeditControl=Selection of Reset will increase slice count due to use of real FFs and instead of SRLs  en=off  latency=5  reg_retiming=on  dbl_ovrd=off  block_type=delay
  Delay1 : xbsIndex_r4/Delay  rst=off  infoeditControl=Selection of Reset will increase slice count due to use of real FFs and instead of SRLs  en=off  latency=5  reg_retiming=on  dbl_ovrd=off  block_type=delay
  Delay10 : xbsIndex_r4/Delay  rst=off  infoeditControl=Selection of Reset will increase slice count due to use of real FFs and instead of SRLs  en=off  latency=5  reg_retiming=on  dbl_ovrd=off  block_type=delay
  Mux : xbsIndex_r4/Mux  inputs=8  en=off  latency=1  precision=Full  arith_type=Unsigned  n_bits=16  bin_pt=14  quantization=Truncate  overflow=Wrap  dbl_ovrd=off  block_type=mux
  Register{,1..7} (8 alike) : xbsIndex_r4/Register  init=0  rst=off  en=on  dbl_ovrd=off  block_type=register
  Register{8..14} (7 alike) : xbsIndex_r4/Register  init=0  rst=off  en=off  dbl_ovrd=off  block_type=register
  out : Outport
  wires:
  Register1/1 -> Mux/3
  in/1 -> AddSub/2
  Mux/1 -> out/1
  Delay1/1 -> AddSub1/1
  Delay/1 -> AddSub/1
  Register3/1 -> Mux/5
  AddSub1/1 -> AddSub2/2, Delay1/1
  sync/1 -> Register8/1, Register/2
  AddSub/1 -> AddSub1/2, Delay/1
  Register6/1 -> Mux/8
  Register2/1 -> Mux/4
  Register5/1 -> Mux/7
  Register4/1 -> Mux/6
  Register7/1 -> Mux/9
  sel/1 -> Mux/1
  Register/1 -> Mux/2
  Delay10/1 -> AddSub2/1
  Register8/1 -> Register9/1, Register1/2
  Register9/1 -> Register10/1, Register2/2
  Register10/1 -> Register11/1, Register3/2
  Register11/1 -> Register12/1, Register4/2
  Register12/1 -> Register13/1, Register5/2
  Register13/1 -> Register14/1, Register6/2
  Register14/1 -> Register7/2
  AddSub2/1 -> Register1/1, Register2/1, Register3/1, Register4/1, Register5/1, Register6/1, Register7/1, Register/1, Delay10/1

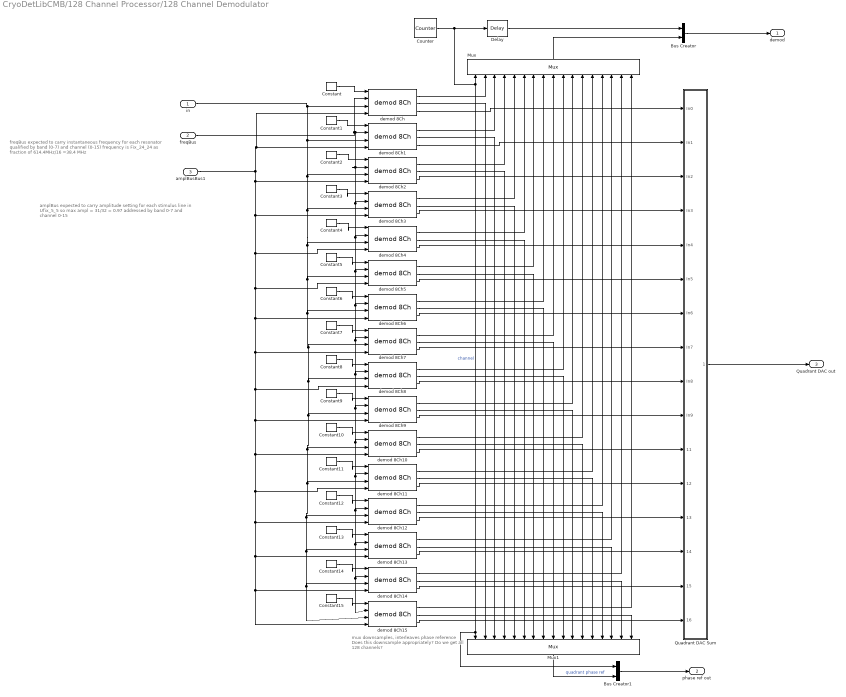
== system CryoDetLibCMB/128 Channel Processor/128 Channel Demodulator ==
  note: amplBus expected to carry  amplitude setting for each stimulus line
      | in Ufix_5_5 so max ampl = 31/32 = 0.97
      | addressed by band 0-7 and channel 0-15
  note: freqBus expected to carry instantaneous frequency for each resonator
      | qualified by band (0-7) and channel (0-15)
      | frequency is Fix_24_24 as fraction of 614.4MHz/16 =38.4 MHz
  note: mux downsamples, interleaves phase reference
      | Does this downsample appropriately?
      | Do we get all 128 channels?
  in : Inport
  freqBus : Inport  Port=2
  amplBusBus1 : Inport  Port=3
  Bus Creator : BusCreator  Inputs=2
  Bus Creator1 : BusCreator  Inputs=2
  Constant : xbsIndex_r4/Constant  const=0  gui_display_data_type=Fixed-point  arith_type=Unsigned  n_bits=4  bin_pt=0  preci_type=Single  exp_width=8  frac_width=24  explicit_period=off  period=1  equ=P=C  opselect=C  inp2=PCIN>>17  opr=+  inp1=P  carry=CIN  dbl_ovrd=off  block_type=constant
  Constant1 : xbsIndex_r4/Constant  const=1  gui_display_data_type=Fixed-point  arith_type=Unsigned  n_bits=4  bin_pt=0  preci_type=Single  exp_width=8  frac_width=24  explicit_period=off  period=1  equ=P=C  opselect=C  inp2=PCIN>>17  opr=+  inp1=P  carry=CIN  dbl_ovrd=off  block_type=constant
  Constant10 : xbsIndex_r4/Constant  const=10  gui_display_data_type=Fixed-point  arith_type=Unsigned  n_bits=4  bin_pt=0  preci_type=Single  exp_width=8  frac_width=24  explicit_period=off  period=1  equ=P=C  opselect=C  inp2=PCIN>>17  opr=+  inp1=P  carry=CIN  dbl_ovrd=off  block_type=constant
  Constant11 : xbsIndex_r4/Constant  const=11  gui_display_data_type=Fixed-point  arith_type=Unsigned  n_bits=4  bin_pt=0  preci_type=Single  exp_width=8  frac_width=24  explicit_period=off  period=1  equ=P=C  opselect=C  inp2=PCIN>>17  opr=+  inp1=P  carry=CIN  dbl_ovrd=off  block_type=constant
  Constant12 : xbsIndex_r4/Constant  const=12  gui_display_data_type=Fixed-point  arith_type=Unsigned  n_bits=4  bin_pt=0  preci_type=Single  exp_width=8  frac_width=24  explicit_period=off  period=1  equ=P=C  opselect=C  inp2=PCIN>>17  opr=+  inp1=P  carry=CIN  dbl_ovrd=off  block_type=constant
  Constant13 : xbsIndex_r4/Constant  const=13  gui_display_data_type=Fixed-point  arith_type=Unsigned  n_bits=4  bin_pt=0  preci_type=Single  exp_width=8  frac_width=24  explicit_period=off  period=1  equ=P=C  opselect=C  inp2=PCIN>>17  opr=+  inp1=P  carry=CIN  dbl_ovrd=off  block_type=constant
  Constant14 : xbsIndex_r4/Constant  const=14  gui_display_data_type=Fixed-point  arith_type=Unsigned  n_bits=4  bin_pt=0  preci_type=Single  exp_width=8  frac_width=24  explicit_period=off  period=1  equ=P=C  opselect=C  inp2=PCIN>>17  opr=+  inp1=P  carry=CIN  dbl_ovrd=off  block_type=constant
  Constant15 : xbsIndex_r4/Constant  const=15  gui_display_data_type=Fixed-point  arith_type=Unsigned  n_bits=4  bin_pt=0  preci_type=Single  exp_width=8  frac_width=24  explicit_period=off  period=1  equ=P=C  opselect=C  inp2=PCIN>>17  opr=+  inp1=P  carry=CIN  dbl_ovrd=off  block_type=constant
  Constant2 : xbsIndex_r4/Constant  const=2  gui_display_data_type=Fixed-point  arith_type=Unsigned  n_bits=4  bin_pt=0  preci_type=Single  exp_width=8  frac_width=24  explicit_period=off  period=1  equ=P=C  opselect=C  inp2=PCIN>>17  opr=+  inp1=P  carry=CIN  dbl_ovrd=off  block_type=constant
  Constant3 : xbsIndex_r4/Constant  const=3  gui_display_data_type=Fixed-point  arith_type=Unsigned  n_bits=4  bin_pt=0  preci_type=Single  exp_width=8  frac_width=24  explicit_period=off  period=1  equ=P=C  opselect=C  inp2=PCIN>>17  opr=+  inp1=P  carry=CIN  dbl_ovrd=off  block_type=constant
  Constant4 : xbsIndex_r4/Constant  const=4  gui_display_data_type=Fixed-point  arith_type=Unsigned  n_bits=4  bin_pt=0  preci_type=Single  exp_width=8  frac_width=24  explicit_period=off  period=1  equ=P=C  opselect=C  inp2=PCIN>>17  opr=+  inp1=P  carry=CIN  dbl_ovrd=off  block_type=constant
  Constant5 : xbsIndex_r4/Constant  const=5  gui_display_data_type=Fixed-point  arith_type=Unsigned  n_bits=4  bin_pt=0  preci_type=Single  exp_width=8  frac_width=24  explicit_period=off  period=1  equ=P=C  opselect=C  inp2=PCIN>>17  opr=+  inp1=P  carry=CIN  dbl_ovrd=off  block_type=constant
  Constant6 : xbsIndex_r4/Constant  const=6  gui_display_data_type=Fixed-point  arith_type=Unsigned  n_bits=4  bin_pt=0  preci_type=Single  exp_width=8  frac_width=24  explicit_period=off  period=1  equ=P=C  opselect=C  inp2=PCIN>>17  opr=+  inp1=P  carry=CIN  dbl_ovrd=off  block_type=constant
  Constant7 : xbsIndex_r4/Constant  const=7  gui_display_data_type=Fixed-point  arith_type=Unsigned  n_bits=4  bin_pt=0  preci_type=Single  exp_width=8  frac_width=24  explicit_period=off  period=1  equ=P=C  opselect=C  inp2=PCIN>>17  opr=+  inp1=P  carry=CIN  dbl_ovrd=off  block_type=constant
  Constant8 : xbsIndex_r4/Constant  const=8  gui_display_data_type=Fixed-point  arith_type=Unsigned  n_bits=4  bin_pt=0  preci_type=Single  exp_width=8  frac_width=24  explicit_period=off  period=1  equ=P=C  opselect=C  inp2=PCIN>>17  opr=+  inp1=P  carry=CIN  dbl_ovrd=off  block_type=constant
  Constant9 : xbsIndex_r4/Constant  const=9  gui_display_data_type=Fixed-point  arith_type=Unsigned  n_bits=4  bin_pt=0  preci_type=Single  exp_width=8  frac_width=24  explicit_period=off  period=1  equ=P=C  opselect=C  inp2=PCIN>>17  opr=+  inp1=P  carry=CIN  dbl_ovrd=off  block_type=constant
  Counter : xbsIndex_r4/Counter  cnt_type=Free Running  cnt_to=Inf  operation=Up  start_count=0  cnt_by_val=1  arith_type=Unsigned  n_bits=4  bin_pt=0  load_pin=off  rst=off  en=off  explicit_period=on  period=Tclk  use_behavioral_HDL=off  implementation=Fabric  dbl_ovrd=off  block_type=counter
  Delay : xbsIndex_r4/Delay  rst=off  infoeditControl=Selection of Reset will increase slice count due to use of real FFs and instead of SRLs  en=off  latency=1  reg_retiming=off  dbl_ovrd=off  block_type=delay
  Mux : xbsIndex_r4/Mux  inputs=16  en=off  latency=1  precision=Full  arith_type=Unsigned  n_bits=16  bin_pt=14  quantization=Truncate  overflow=Wrap  dbl_ovrd=off  block_type=mux
  Mux1 : xbsIndex_r4/Mux  inputs=16  en=off  latency=1  precision=Full  arith_type=Unsigned  n_bits=16  bin_pt=14  quantization=Truncate  overflow=Wrap  dbl_ovrd=off  block_type=mux
  Quadrant DAC Sum : Subsystem
  demod 8Ch{,1..15} (16 alike) : CryoDetLibCMB/demod 8Ch
  demod : Outport
  phase ref out : Outport  Port=2
  Quadrant DAC out : Outport  Port=3
  wires:
  Constant/1 -> demod 8Ch/1
  Constant1/1 -> demod 8Ch1/1
  Constant2/1 -> demod 8Ch2/1
  Constant3/1 -> demod 8Ch3/1
  Constant4/1 -> demod 8Ch4/1
  Constant5/1 -> demod 8Ch5/1
  Constant6/1 -> demod 8Ch6/1
  Constant7/1 -> demod 8Ch7/1
  Constant8/1 -> demod 8Ch8/1
  Constant9/1 -> demod 8Ch9/1
  Constant10/1 -> demod 8Ch10/1
  Constant11/1 -> demod 8Ch11/1
  Constant12/1 -> demod 8Ch12/1
  Constant13/1 -> demod 8Ch13/1
  Constant14/1 -> demod 8Ch14/1
  freqBus/1 -> demod 8Ch2/2, demod 8Ch5/2, demod 8Ch6/2, demod 8Ch7/2, demod 8Ch8/2, demod 8Ch10/2, demod 8Ch11/2, demod 8Ch12/2, demod 8Ch13/2, demod 8Ch14/2, demod 8Ch15/2, demod 8Ch9/2, demod 8Ch4/2, demod 8Ch3/2, demod 8Ch1/2, demod 8Ch/2
  demod 8Ch/1 -> Mux/2
  Counter/1 -> Delay/1, Bus Creator1/1, Mux1/1, Mux/1  "channel"
  Delay/1 -> Bus Creator/1
  Mux/1 -> Bus Creator/2
  demod 8Ch1/1 -> Mux/3
  demod 8Ch2/1 -> Mux/4
  demod 8Ch3/1 -> Mux/5
  demod 8Ch4/1 -> Mux/6
  demod 8Ch5/1 -> Mux/7
  demod 8Ch/2 -> Mux1/2
  demod 8Ch1/2 -> Mux1/3
  demod 8Ch2/2 -> Mux1/4
  demod 8Ch3/2 -> Mux1/5
  demod 8Ch4/2 -> Mux1/6
  demod 8Ch5/2 -> Mux1/7
  demod 8Ch/3 -> Quadrant DAC Sum/1(In0)
  demod 8Ch1/3 -> Quadrant DAC Sum/2(In1)
  demod 8Ch2/3 -> Quadrant DAC Sum/3(In2)
  demod 8Ch3/3 -> Quadrant DAC Sum/4(In3)
  demod 8Ch4/3 -> Quadrant DAC Sum/5(In4)
  demod 8Ch5/3 -> Quadrant DAC Sum/6(In5)
  demod 8Ch6/3 -> Quadrant DAC Sum/7(In6)
  demod 8Ch7/3 -> Quadrant DAC Sum/8(In7)
  demod 8Ch8/3 -> Quadrant DAC Sum/9(In8)
  demod 8Ch9/3 -> Quadrant DAC Sum/10(In9)
  demod 8Ch10/3 -> Quadrant DAC Sum/11(In10)
  demod 8Ch11/3 -> Quadrant DAC Sum/12(In11)
  demod 8Ch12/3 -> Quadrant DAC Sum/13(In12)
  demod 8Ch13/3 -> Quadrant DAC Sum/14(In13)
  demod 8Ch14/3 -> Quadrant DAC Sum/15(In14)
  Constant15/1 -> demod 8Ch15/1
  demod 8Ch15/3 -> Quadrant DAC Sum/16(In15)
  demod 8Ch15/2 -> Mux1/17
  demod 8Ch14/2 -> Mux1/16
  demod 8Ch13/2 -> Mux1/15
  demod 8Ch6/1 -> Mux/8
  demod 8Ch7/1 -> Mux/9
  demod 8Ch8/1 -> Mux/10
  demod 8Ch9/1 -> Mux/11
  demod 8Ch10/1 -> Mux/12
  demod 8Ch11/1 -> Mux/13
  demod 8Ch12/1 -> Mux/14
  demod 8Ch13/1 -> Mux/15
  demod 8Ch14/1 -> Mux/16
  demod 8Ch15/1 -> Mux/17
  demod 8Ch6/2 -> Mux1/8
  demod 8Ch12/2 -> Mux1/14
  demod 8Ch11/2 -> Mux1/13
  demod 8Ch10/2 -> Mux1/12
  demod 8Ch9/2 -> Mux1/11
  demod 8Ch7/2 -> Mux1/9
  demod 8Ch8/2 -> Mux1/10
  Mux1/1 -> Bus Creator1/2  "quadrant phase ref"
  Bus Creator1/1 -> phase ref out/1
  in/1 -> demod 8Ch/3, demod 8Ch2/3, demod 8Ch6/3, demod 8Ch7/3, demod 8Ch8/3, demod 8Ch10/3, demod 8Ch12/3, demod 8Ch15/3, demod 8Ch14/3, demod 8Ch13/3, demod 8Ch11/3, demod 8Ch9/3, demod 8Ch5/3, demod 8Ch4/3, demod 8Ch3/3, demod 8Ch1/3
  Bus Creator/1 -> demod/1
  Quadrant DAC Sum/1(Out2) -> Quadrant DAC out/1
  amplBusBus1/1 -> demod 8Ch/4, demod 8Ch1/4, demod 8Ch4/4, demod 8Ch5/4, demod 8Ch6/4, demod 8Ch7/4, demod 8Ch8/4, demod 8Ch9/4, demod 8Ch10/4, demod 8Ch11/4, demod 8Ch12/4, demod 8Ch13/4, demod 8Ch14/4, demod 8Ch15/4, demod 8Ch3/4, demod 8Ch2/4

== system CryoDetLibCMB/128 Channel Processor/Loop Filter ==
  In1 : Inport
  Out1 : Outport
  wires:
  In1/1 -> Out1/1

== system CryoDetLibCMB/128 Channel Processor/dF ==
  demod in : Inport
  phase ref in : Inport  Port=2
  Out1 : Outport
  wires:
  demod in/1 -> Out1/1
